simulink model "RateAdaptivity"  (R2020a)
settings: Solver=FixedStepAuto  StartTime=0.0  StopTime=10.0  FixedStep=1e-3  RelTol=1e-3  EnableMultiTasking=on
libraries: frdmk64flib x4
settings Model: ExtModeTrigDuration=5  Creator=theodor  LastModifiedBy=theodor
settings OptimizationCC: BlockReduction=off  DefaultParameterBehavior=Inlined  BufferReuse=off  EnhancedBackFolding=on  PassReuseOutputArgsAs=Individual arguments  ZeroExternalMemoryAtStartup=off  ZeroInternalMemoryAtStartup=off  MaxStackSize=64  OptimizeBlockOrder=speed  DifferentSizesBufferReuse=on  EfficientTunableParamExpr=on
settings DebuggingCC: ParameterTunabilityLossMsg=error
settings HardwareCC: ProdBitPerPointer=32  ProdBitPerSizeT=32  ProdBitPerPtrDiffT=32  ProdLargestAtomicInteger=Long  ProdLargestAtomicFloat=Double  ProdWordSize=32  ProdHWDeviceType=ARM Compatible->ARM Cortex
settings SFSimCC: MATLABDynamicMemAlloc=off
settings RTWCC: SystemTargetFile=ert.tlc  HardwareBoard=NXP FRDM-K64F  TemplateMakefile=ert_default_tmf  Toolchain=GNU Tools for ARM Embedded Processors
settings CodeAppCC: ForceParamTrailComments=on  IgnoreCustomStorageClasses=off  OperatorAnnotations=on  SimulinkDataObjDesc=on  SFDataObjDesc=on  InsertBlockDesc=on

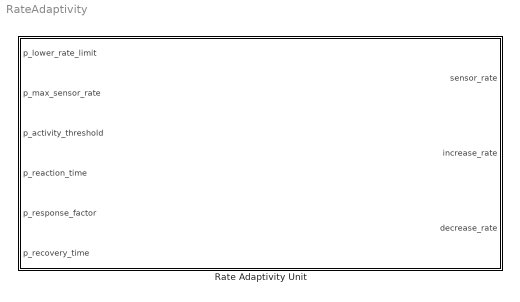
== system RateAdaptivity ==
  Rate Adaptivity Unit : Subsystem

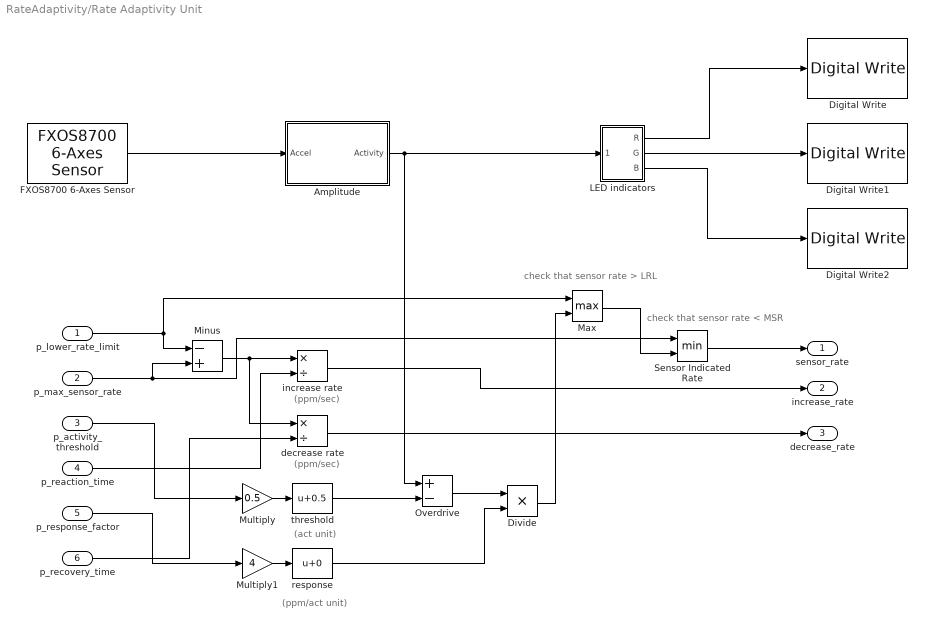
== system RateAdaptivity/Rate Adaptivity Unit ==
  note: check that sensor rate < MSR
  note: check that sensor rate > LRL
  note: (ppm/act unit)
  note: (act unit)
  note: (ppm/sec)
  note: (ppm/sec)
  p_lower_rate_limit : Inport
  p_max_sensor_rate : Inport  Port=2
  p_activity_threshold : Inport  Port=3
  p_reaction_time : Inport  Port=4
  p_response_factor : Inport  Port=5
  p_recovery_time : Inport  Port=6
  Amplitude : Subsystem
  Digital Write : frdmk64flib/Digital Write  Whichpin=RED_LED
  Digital Write1 : frdmk64flib/Digital Write  Whichpin=GREEN_LED
  Digital Write2 : frdmk64flib/Digital Write  Whichpin=BLUE_LED
  Divide : Product  Inputs=**
  FXOS8700 6-Axes Sensor : frdmk64flib/FXOS8700 6-Axes Sensor  Activesensor=Accelerometer only  ODR=100Hz  HybridODR=100Hz  Accelfullrange=-4g to +4g  SampleTime=-1
  LED indicators : Subsystem
  Max : MinMax  Function=max  Inputs=2
  Minus : Sum  Inputs=-+
  Multiply : Gain  Gain=0.5
  Multiply1 : Gain  Gain=4
  Overdrive : Sum  Inputs=+-
  Sensor Indicated Rate : MinMax  Inputs=2
  decrease rate : Product  Inputs=*/
  increase rate : Product  Inputs=*/
  response : Bias
  threshold : Bias  Bias=0.5
  sensor_rate : Outport
  increase_rate : Outport  Port=2
  decrease_rate : Outport  Port=3
  wires:
  LED indicators/3(B) -> Digital Write2/1
  LED indicators/2(G) -> Digital Write1/1
  LED indicators/1(R) -> Digital Write/1
  FXOS8700 6-Axes Sensor/1 -> Amplitude/1(Accel)
  Amplitude/1(Activity) -> Overdrive/1, LED indicators/1(input)
  p_lower_rate_limit/1 -> Max/1, Minus/1
  p_max_sensor_rate/1 -> Minus/2, Sensor Indicated Rate/1
  Minus/1 -> decrease rate/1, increase rate/1
  p_reaction_time/1 -> increase rate/2
  p_recovery_time/1 -> decrease rate/2
  Multiply/1 -> threshold/1
  p_activity_threshold/1 -> Multiply/1
  Multiply1/1 -> response/1
  p_response_factor/1 -> Multiply1/1
  Max/1 -> Sensor Indicated Rate/2
  threshold/1 -> Overdrive/2
  response/1 -> Divide/2
  Overdrive/1 -> Divide/1
  Divide/1 -> Max/2
  Sensor Indicated Rate/1 -> sensor_rate/1
  increase rate/1 -> increase_rate/1
  decrease rate/1 -> decrease_rate/1

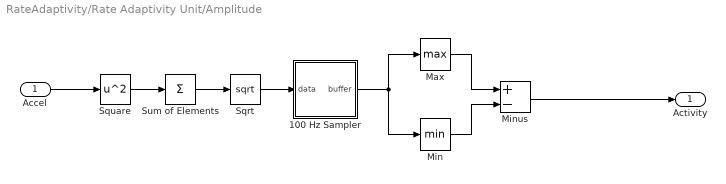
== system RateAdaptivity/Rate Adaptivity Unit/Amplitude ==
  Accel : Inport
  100 Hz Sampler : Stateflow chart  TreatAsAtomicUnit=on
  Max : MinMax  Function=max
  Min : MinMax
  Minus : Sum  Inputs=+-
  Sqrt : Sqrt  SaturateOnIntegerOverflow=on
  Square : Math  Operator=square  SaturateOnIntegerOverflow=on
  Sum of Elements : Sum  Inputs=+
  Activity : Outport
  wires:
  Square/1 -> Sum of Elements/1
  Sum of Elements/1 -> Sqrt/1
  Sqrt/1 -> 100 Hz Sampler/1(data)
  Min/1 -> Minus/2
  Minus/1 -> Activity/1
  Accel/1 -> Square/1
  Max/1 -> Minus/1
  100 Hz Sampler/1(buffer) -> Min/1, Max/1

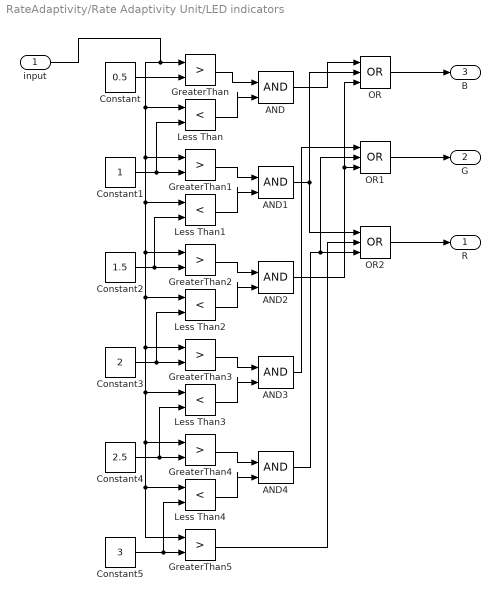
== system RateAdaptivity/Rate Adaptivity Unit/LED indicators ==
  input : Inport
  AND{,1..4} (5 alike) : Logic  IconShape=distinctive  AllPortsSameDT=off  OutDataTypeStr=boolean
  Constant : Constant  Value=0.5
  Constant1 : Constant
  Constant2 : Constant  Value=1.5
  Constant3 : Constant  Value=2
  Constant4 : Constant  Value=2.5
  Constant5 : Constant  Value=3
  GreaterThan{,1..5} (6 alike) : RelationalOperator  Operator=>  OutDataTypeStr=boolean  RndMeth=Simplest
  Less Than{,1..4} (5 alike) : RelationalOperator  Operator=<  OutDataTypeStr=boolean  RndMeth=Simplest
  OR : Logic  Operator=OR  Inputs=3  IconShape=distinctive  AllPortsSameDT=off  OutDataTypeStr=boolean
  OR1 : Logic  Operator=OR  Inputs=3  IconShape=distinctive  AllPortsSameDT=off  OutDataTypeStr=boolean
  OR2 : Logic  Operator=OR  Inputs=3  IconShape=distinctive  AllPortsSameDT=off  OutDataTypeStr=boolean
  R : Outport
  G : Outport  Port=2
  B : Outport  Port=3
  wires:
  OR1/1 -> G/1
  Less Than4/1 -> AND4/2
  Less Than/1 -> AND/2
  Constant/1 -> GreaterThan/2
  AND1/1 -> OR2/1, OR/2
  OR/1 -> B/1
  AND4/1 -> OR1/2, OR2/3
  GreaterThan1/1 -> AND1/1
  Less Than3/1 -> AND3/2
  OR2/1 -> R/1
  AND/1 -> OR/1
  Constant2/1 -> Less Than1/2, GreaterThan2/2
  AND3/1 -> OR1/1
  GreaterThan5/1 -> OR2/2
  Constant5/1 -> Less Than4/2, GreaterThan5/2
  Constant1/1 -> Less Than/2, GreaterThan1/2
  input/1 -> GreaterThan/1, Less Than/1, GreaterThan1/1, Less Than1/1, GreaterThan2/1, Less Than2/1, GreaterThan3/1, Less Than3/1, GreaterThan4/1, Less Than4/1, GreaterThan5/1
  GreaterThan3/1 -> AND3/1
  GreaterThan2/1 -> AND2/1
  GreaterThan/1 -> AND/1
  Less Than2/1 -> AND2/2
  AND2/1 -> OR1/3, OR/3
  Less Than1/1 -> AND1/2
  Constant4/1 -> Less Than3/2, GreaterThan4/2
  Constant3/1 -> Less Than2/2, GreaterThan3/2
  GreaterThan4/1 -> AND4/1

== stateflow chart RateAdaptivity/Rate Adaptivity Unit/Amplitude/100 Hz Sampler ==
  state SAMPLE
    entry:
    buffer(2:50) = buffer(1:49);
    buffer(1) = data;
  (default) -> SAMPLE
  SAMPLE -> SAMPLE : after(10,msec)
  data: data input; buffer output size=50 =zeros(50,1)
